simulink model "Non_linear_observers"  (R2017a)
settings: Solver=VariableStepAuto  StartTime=0.0  StopTime=10.0  RelTol=1e-3
values from neighbouring files (symbols this model uses):
  A = [0 1;0 0]    [Adaptive_Control.m]    (also in Adaptive_Control_Linear.m = [0 1;a1 a2]; HGO.m = [0 1;-1 -1]; Non_linear_observers_.m; feedback-integrator.m = [1 1;0 0])
  B = [0;1]    [Adaptive_Control.m]    (also in Adaptive_Control_Linear.m = [0;b]; Non_linear_observers_.m; feedback-integrator.m = [0;1+b]; mini_projet.m = [0;1+b])
  C = [1 0]    [Adaptive_Control.m]    (also in Adaptive_Control_Linear.m; HGO.m; Non_linear_observers_.m; feedback-integrator.m)
  D = 0    [Non_linear_observers_.m]    (also in feedback-integrator.m; mini_projet.m)
  L = [3 1]'    [Non_linear_observers_.m]    (also in projet_AAV.m = 1; testing_linear_observer.m = L')
settings Model: Creator=firass2019  LastModifiedBy=firass2019

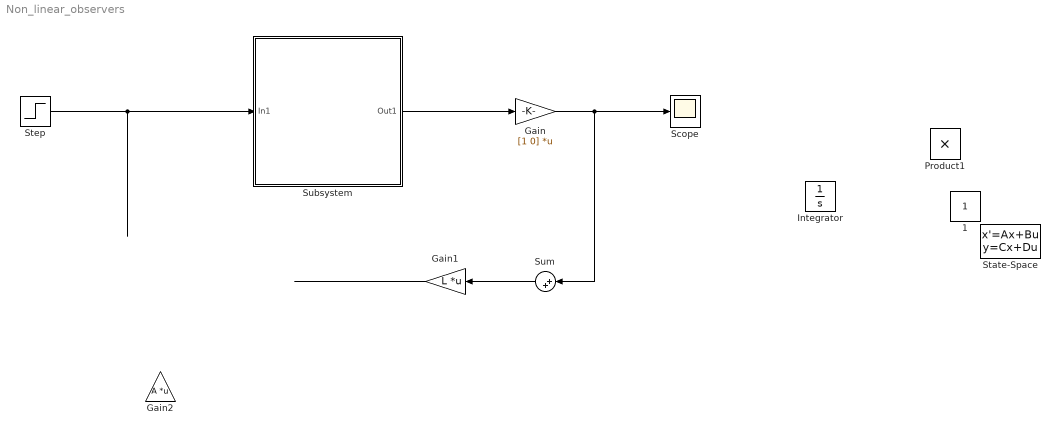
== system Non_linear_observers ==
  1 : Constant
  Gain : Gain  Gain=[1 0]  Multiplication=Matrix(K*u)
  Gain1 : Gain  Gain=L  Multiplication=Matrix(K*u)
  Gain2 : Gain  Gain=A  Multiplication=Matrix(K*u)
  Integrator : Integrator  InitialCondition=0.1
  Product1 : Product
  Scope : Scope
  State-Space : StateSpace  A=A  B=B  C=C  D=D  X0=0
  Step : Step  Time=0  After=0  SampleTime=0
  Subsystem : Subsystem
  Sum : Sum  Inputs=|++
  wires:
  Step/1 -> Subsystem/1(In1)
  Subsystem/1(Out1) -> Gain/1
  Gain/1 -> Sum/1, Scope/1
  ? -> Sum/2
  Sum/1 -> Gain1/1
  Gain1/1 -> ?

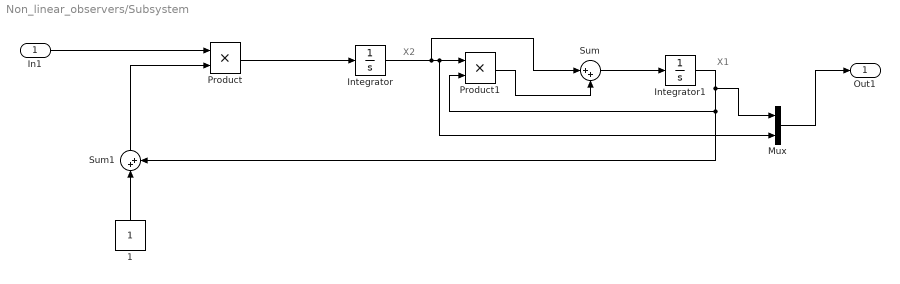
== system Non_linear_observers/Subsystem ==
  note: X2
  note: X1
  In1 : Inport
  1 : Constant
  Integrator : Integrator  InitialCondition=0.1
  Integrator1 : Integrator
  Mux : Mux  Inputs=2
  Product : Product
  Product1 : Product
  Sum : Sum  Inputs=|++
  Sum1 : Sum  Inputs=|++
  Out1 : Outport
  wires:
  Integrator1/1 -> Mux/1, Product1/2, Sum1/2
  Product1/1 -> Sum/2
  Sum1/1 -> Product/2
  In1/1 -> Product/1
  Product/1 -> Integrator/1
  1/1 -> Sum1/1
  Integrator/1 -> Sum/1, Mux/2, Product1/1
  Sum/1 -> Integrator1/1
  Mux/1 -> Out1/1
